simulink model "test_memory"  (Simulink 7.6)
settings: Solver=FixedStepDiscrete  StartTime=0.0  StopTime=10  FixedStep=.1  RelTol=1e-3
settings Model: Creator=Thing 1  LastModifiedBy=Administrator
settings RTWCC: TargetLang=C++

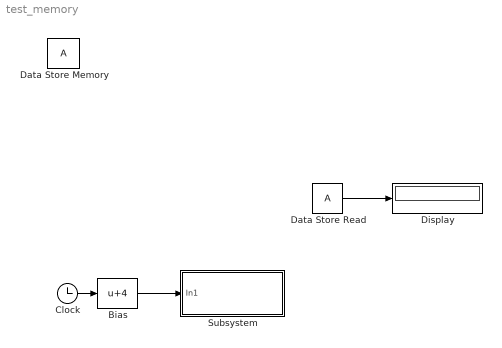
== system test_memory ==
  Bias : Bias  Bias=4
  Clock : Clock
      settings: Decimation=10
  Data Store Memory : DataStoreMemory  ReadBeforeWriteMsg=warning  WriteAfterWriteMsg=warning  WriteAfterReadMsg=warning
  Data Store Read : DataStoreRead
  Display : Display
      settings: Decimation=5
  Subsystem : Subsystem
  wires:
  Data Store Read/1 -> Display/1
  Clock/1 -> Bias/1
  Bias/1 -> Subsystem/1(In1)

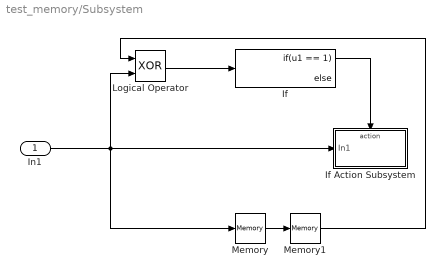
== system test_memory/Subsystem ==
  In1 : Inport
  If : If  IfExpression=u1 == 1
  If Action Subsystem : Subsystem  TreatAsAtomicUnit=on
  Logical Operator : Logic  Operator=XOR  AllPortsSameDT=off  OutDataTypeStr=boolean
  Memory : Memory
  Memory1 : Memory
  wires:
  In1/1 -> If Action Subsystem/1(In1), Memory/1, Logical Operator/2
  Logical Operator/1 -> If/1
  If/1 -> If Action Subsystem/Action
  Memory/1 -> Memory1/1
  Memory1/1 -> Logical Operator/1

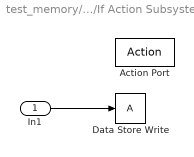
== system test_memory/Subsystem/If Action Subsystem ==
  In1 : Inport
  Action Port : ActionPort  ActionType=then
  Data Store Write : DataStoreWrite
  wires:
  In1/1 -> Data Store Write/1
